simulink model "GraduatedPotentials"  (Simulink 8.4)
settings: Solver=ode45  StartTime=0.0  StopTime=1  RelTol=1e-3
libraries: NeuroModelerLibrary x5
settings Model: Creator=Tim  LastModifiedBy=Tim
settings OptimizationCC: InitFltsAndDblsToZero=on

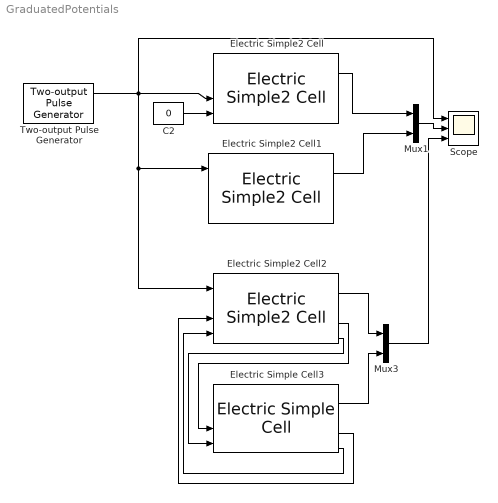
== system GraduatedPotentials ==
  C2 : Constant  Value=0
  Electric Simple Cell3 : NeuroModelerLibrary/Simple Cells/Electric Simple Cell
      link override LTZone: T=2
  Electric Simple2 Cell : NeuroModelerLibrary/Simple Cells/Electric Simple2 Cell
      link override LTZone: T=2
  Electric Simple2 Cell1 : NeuroModelerLibrary/Simple Cells/Electric Simple2 Cell
      link override LTZone: T=2
  Electric Simple2 Cell2 : NeuroModelerLibrary/Simple Cells/Electric Simple2 Cell
      link override LTZone: T=2
  Mux1 : Mux  Inputs=2
  Mux3 : Mux  Inputs=2
  Scope : Scope  NumInputPorts=3
      settings: YMin=0~-0.005~0  YMax=1~0.03~0.075
  Two-output Pulse Generator : NeuroModelerLibrary/Support/Two-output Pulse Generator  A=1  P1=50  P2=50  PW=1  ST=0.001  OOn1=0.2  OOff1=0.8  OOn2=0.2  OOff2=0.8
  wires:
  C2/1 -> Electric Simple2 Cell/4
  Two-output Pulse Generator/1 -> Scope/1, Electric Simple2 Cell/3, Electric Simple2 Cell1/1, Electric Simple2 Cell2/1
  Mux1/1 -> Scope/2
  Electric Simple2 Cell/2 -> Mux1/1
  Electric Simple2 Cell1/2 -> Mux1/2
  Electric Simple2 Cell2/2 -> Mux3/1
  Electric Simple Cell3/2 -> Mux3/2
  Electric Simple2 Cell2/4 -> Electric Simple Cell3/3
  Electric Simple2 Cell2/5 -> Electric Simple Cell3/4
  Mux3/1 -> Scope/3
  Electric Simple Cell3/4 -> Electric Simple2 Cell2/3
  Electric Simple Cell3/5 -> Electric Simple2 Cell2/4
